simulink model "flux_linkage"  (R2020b)
settings: Solver=VariableStepAuto  StartTime=0.0  StopTime=1  RelTol=1e-3
InitFcn:
  | Rs=0.43;
  | 
  | Lls=0.002
  | 
  | Rr=0.816;
  | 
  | Llr=0.002
  | 
  | Lm=0.6931;
  | 
  | 
  | J=0.085;
  | np=2;
  | 
  | Ts=1e-5;
  | 
  | Udc=600*sqrt(3)
  | Tpwm = 4e-4;
  | 
  | Udc = 2700
  | J = 0.1
  | Llr = 0.006
  | Lls = 0.00116
  | Lm = 0.0254
  | Rr = 0.16
  | Rs = 0.15
  | 
  | Ls = 1.5*Lm+Lls
  | Lr = 1.5*Lm+Llr
  | Tr = Lr/Rr;
  | sigma = (Ls*Lr-Lm*Lm)/Ls/Lr;
model workspace (MAT data in the model file):
  Tsys = 2e-06
  sample_time = 1e-06
libraries: powerlib x17, simulink x3
settings Model: SimulationMode=accelerator  OrderedModelArguments=off  Creator=messer  LastModifiedBy=messer

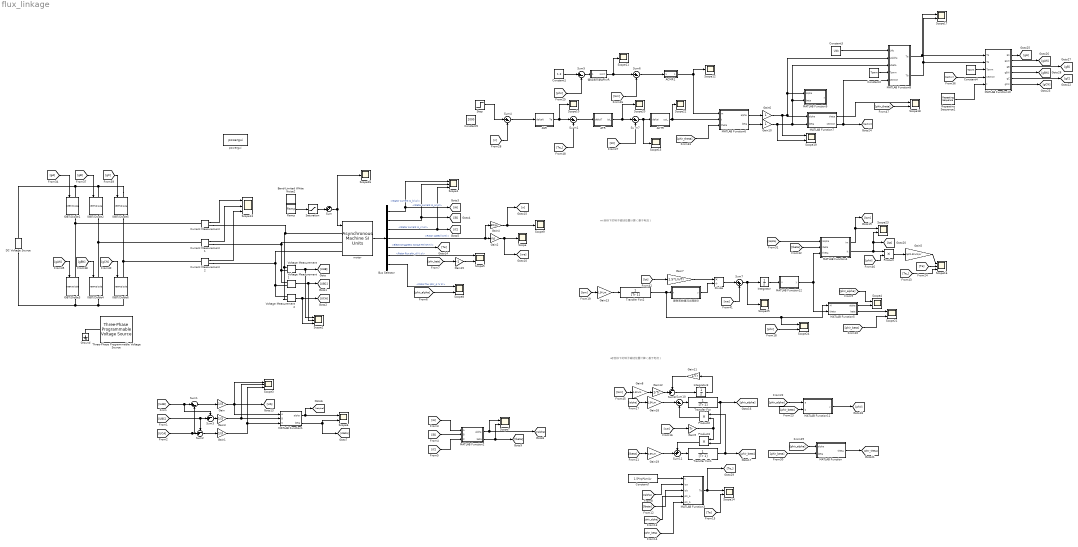
== system flux_linkage ==
  note: αβ坐标下的转子磁链位置计算（基于电流）
  note: mt坐标下的转子磁链位置计算（基于电流）
  ACMR1 : Subsystem
  ACTR : Subsystem
  ASR : Subsystem
  ATR : Subsystem
  Band-Limited White Noise2 : simulink/Sources/Band-Limited White Noise  Cov=[0.0001]  Ts=1e-4  seed=[130341]
  Bus Selector : BusSelector  OutputSignals=Stator measurements.Stator current is_a (A),Stator measurements.Stator current is_b (A),Stator measurements.Stator current is_c (A),Mechanical.Rotor speed (wm),Mechanical.Electromagnetic torque Te (N*m),Rotor measurements.Rotor flux phir_d (V s),Rotor measurements.Rotor flux phir_q (V s)
  Constant1 : Constant  Value=1.2
  Constant2 : Constant  Value=Tpwm
  Constant3 : Constant  Value=Udc
  Constant4 : Constant  Value=Tpwm
  Constant5 : Constant  Value=2000
  Constant7 : Constant  Value=1.5*np*Lm/Lr
  Current Measurement : powerlib/Measurements/Current Measurement  PhasorSimulation=off  OutputType=Complex  PSBequivalent=0
  Current Measurement1 : powerlib/Measurements/Current Measurement  PhasorSimulation=off  OutputType=Complex  PSBequivalent=0
  Current Measurement2 : powerlib/Measurements/Current Measurement  PhasorSimulation=off  OutputType=Complex  PSBequivalent=0
  DC Voltage Source : powerlib/Electrical Sources/DC Voltage Source  Amplitude=Udc  Measurements=None
  Divide : Product  Inputs=*/
  Gain : Gain  Gain=1/3
  Gain1 : Gain  Gain=1/3
  Gain10 : Gain
  Gain11 : Gain  Gain=1/Tr
  Gain12 : Gain  Gain=1/Tr
  Gain{8,13,18..19} (4 alike) : Gain  Gain=1.5*Lm
  Gain15 : Gain  Gain=-1
  Gain2 : Gain  Gain=np
  Gain3 : Gain  Gain=1/3
  Gain4 : Gain  Gain=30/pi
  Gain5 : Gain  Gain=np*1.5*Lm/Lr
  Gain6 : Gain
  Gain7 : Gain  Gain=1.5*Lm/Tr
  Gain9 : Gain  Gain=Tr
  Ground : powerlib/Elements/Ground  LConnTagsString=a
  IGBT/Diode{1..6} (6 alike) : powerlib/Power Electronics/IGBT//Diode  Ron=1e-3  Rs=1e5  Cs=inf  Measurements=on
  Integrator : Integrator  InitialCondition=1e-5
  Integrator3 : Integrator  InitialCondition=1e-5
  MATLAB Function : MATLAB Function  TreatAsAtomicUnit=on
  MATLAB Function1 : MATLAB Function  TreatAsAtomicUnit=on
  MATLAB Function10 : MATLAB Function  TreatAsAtomicUnit=on
  MATLAB Function11 : MATLAB Function  TreatAsAtomicUnit=on
  MATLAB Function12 : MATLAB Function  TreatAsAtomicUnit=on
  MATLAB Function2 : MATLAB Function  TreatAsAtomicUnit=on
  MATLAB Function3 : MATLAB Function  TreatAsAtomicUnit=on
  MATLAB Function4 : MATLAB Function  TreatAsAtomicUnit=on
  MATLAB Function5 : MATLAB Function  TreatAsAtomicUnit=on
  MATLAB Function6 : MATLAB Function  TreatAsAtomicUnit=on
  MATLAB Function7 : MATLAB Function  TreatAsAtomicUnit=on
  MATLAB Function8 : MATLAB Function  TreatAsAtomicUnit=on
  MATLAB Function9 : MATLAB Function  TreatAsAtomicUnit=on
  Product : Product
  Product2 : Product
  Product3 : Product
  Ramp : simulink/Sources/Ramp  slope=100  start=0.15  InitialOutput=5
  Repeating Sequence1 : simulink/Sources/Repeating Sequence  rep_seq_t=[0 Tpwm]  rep_seq_y=[0 Tpwm]
  Saturation : Saturate  UpperLimit=20  LowerLimit=0
  Scope{,9..12,15,20,22,25..26} (10 alike) : Scope
  Scope{1..3,13,16} (5 alike) : Scope  NumInputPorts=3
  Scope{4..8,14,17..19,21,23..24} (12 alike) : Scope  NumInputPorts=2
  Step : Step  Time=0.5  Before=2000  After=3000  SampleTime=0
  Su`m1 : Sum  Inputs=|+-
  Su`m7 : Sum  Inputs=|+-
  Sum : Sum  Inputs=++|
  Sum{1,4..6,10} (5 alike) : Sum  Inputs=|+-
  Sum11 : Sum  Inputs=++|
  Sum2 : Sum  Inputs=-+|
  Sum3 : Sum  Inputs=-+|
  Sum7 : Sum  Inputs=|++
  Sum8 : Sum  Inputs=-+|
  Three-Phase Programmable Voltage Source : powerlib/Electrical Sources/Three-Phase Programmable Voltage Source  PositiveSequence="[380/sqrt(2)  0 50]"  VariationEntity=None  VariationType=Table of time-amplitude pairs  VariationTypeAlt=Step  VariationStep=0.5  VariationRate=10  VariationMagnitude=0.3  VariationFrequency=2  VariationTiming=[1 2]  VariationPhaseA=off  Amplitudes=[1 0.8 1.2 1.0]  TimeValues=[0 0.1 0.15 0.2]  HarmonicGeneration=off  HarmonicA=[3 0.2 -25 0]  HarmonicB=[2 0.15 35 2]  Timing="[0.05  3]"  BusType=swing  Pref=0  Qref=0  Qmin=-inf  Qmax=inf
  Transfer Fcn : TransferFcn  Denominator=[Tr 1]
  Transfer Fcn1 : TransferFcn  Denominator=[Tr 1]
  Transfer Fcn2 : TransferFcn  Denominator=[Tr 1]
  Voltage Measurement : powerlib/Measurements/Voltage Measurement  PhasorSimulation=off  OutputType=Complex  PSBequivalent=0
  Voltage Measurement1 : powerlib/Measurements/Voltage Measurement  PhasorSimulation=off  OutputType=Complex  PSBequivalent=0
  Voltage Measurement2 : powerlib/Measurements/Voltage Measurement  PhasorSimulation=off  OutputType=Complex  PSBequivalent=0
  motor : powerlib/Machines/Asynchronous Machine SI Units  RotorType=Squirrel-cage  PresetModel=No  MechanicalLoad=Torque Tm  ShowDetailedParameters=on  ReferenceFrame=Stationary  Units=SI  MeasurementBus=off  NominalParameters=[562000 2750 135]  Stator=[Rs Lls]  Rotor=[Rr Llr]  Cage1=[0.4155 0.002066]  Cage2=[0.4168 0.0003495]  Lm=Lm  Mechanical=[J 0 np]  PolePairs=2  InitialConditions=[1 0 0 0 0 0 0 0]  SimulateSaturation=off  Saturation=[14.03593122, 27.81365428, 53.79336849, 72.68890987, 97.98006896, 148.6815601, 215.7428561, 302.9841135, 428.7778367 ; 230, 322, 414, 460, 506, 552, 598, 644, 690]  LoadFlowParameters=1492000  TsPowergui=0  TsBlock=-1  IterativeModel=Trapezoidal non iterative  IterativeDiscreteModel=Trapezoidal non iterative  Pmec=1.492e+006
  powergui : powerlib/powergui  Priority=1  SimulationMode=Discrete  SampleTime=Tsys  frequency=60  Iterations=50  frequencyindice=0  Pbase=100e6  ErrMax=1e-4  UnitsV=kV  UnitsW=MW  buscounter=0  FunctionMessages=off  echomessages=off  EnableUseOfTLC=off  CurrentSourceSwitches=off  DisableSnubberDevices=off  DisableRonSwitches=off  DisableVfSwitches=off  DisplayEquations=off  AutomaticDiscreteSolvers=off  SolverType=Tustin/Backward Euler (TBE)  Interpol=off  ExternalGateDelay=off  methode=off  Ts=100  x0status=blocks  SPID=on  SwTol=0  HookPort=off  NonlinearTolerance=1e-4  nMaxIteration=100  ContinueOnMaxIteration=off  RestoreLinks=warning  ResistiveCurrentMeasurement=off  Frange=[0:2:500]  Ylog=off  Xlog=on  ShowGrid=off  save=off  variable=ZData  structure=0  ZoomFFT=off  StartTime=0.0  cycles=1  DisplayStyle=1  fundamental=60  FreqAxis=off  MaxFrequency=1000  frequencyindicesteady=1  RmsSteady=1  display=off
  磁链调节器APhirR : Subsystem
  避免初始情况出现除0 : MATLAB Function  TreatAsAtomicUnit=on
  wires:
  Bus Selector/4 -> Gain4/1, Gain2/1  "<Rotor speed (wm)>"
  Bus Selector/2 -> Scope1/2, [iB]  "<Stator current is_b (A)>"
  Bus Selector/5 -> [Te]  "<Electromagnetic torque Te (N*m)>"
  Saturation/1 -> Sum/2
  Bus Selector/1 -> [iA], Scope1/1  "<Stator current is_a (A)>"
  motor/1 -> Bus Selector/1
  Bus Selector/3 -> Scope1/3, [iC]  "<Stator current is_c (A)>"
  Ramp/1 -> Saturation/1
  Voltage Measurement1/1 -> [UBC], Scope2/2
  Voltage Measurement/1 -> Scope2/1, [UAB]
  Voltage Measurement2/1 -> [UCA], Scope2/3
  [UAB] -> Sum3/1, Sum1/1
  [UCA] -> Sum1/2, Sum2/2
  Sum1/1 -> Gain/1
  [UBC] -> Sum2/1, Sum3/2
  Sum2/1 -> Gain1/1
  Sum3/1 -> Gain3/1
  Gain3/1 -> MATLAB Function1/2(B), Scope3/2
  Gain/1 -> MATLAB Function1/1(A), [UA], Scope3/1
  Gain1/1 -> MATLAB Function1/3(C), Scope3/3
  Sum/1 -> Scope26/1, motor/1
  MATLAB Function1/1(alpha) -> [Ualpha], Scope6/1
  MATLAB Function1/2(beta) -> [Ubeta], Scope6/2
  MATLAB Function2/2(beta) -> [Ibeta], Scope7/2
  [iB] -> MATLAB Function2/2(B)
  MATLAB Function2/1(alpha) -> Scope7/1, [Ialpha]
  [phir_alpha] -> Scope8/2
  [phir_beta] -> Gain15/1
  Gain15/1 -> Scope5/2
  Bus Selector/6 -> Scope5/1  "<Rotor flux phir_d (V s)>"
  Bus Selector/7 -> Scope8/1  "<Rotor flux phir_q (V s)>"
  Gain2/1 -> [we], Scope/1
  [iA] -> MATLAB Function2/1(A)
  [iC] -> MATLAB Function2/3(C)
  Constant7/1 -> MATLAB Function3/1(c)
  [Ialpha] -> MATLAB Function3/2(isa)
  [Ibeta] -> MATLAB Function3/3(isb)
  [phir_alpha] -> MATLAB Function3/4(phi_a)
  [phir_beta] -> MATLAB Function3/5(phi_b)
  MATLAB Function3/1(Te) -> [Te_], Scope14/1
  [Te] -> Scope14/2
  Gain4/1 -> [n], Scope9/1
  Current Measurement1/1 -> Scope13/2
  Current Measurement2/1 -> Scope13/3
  Current Measurement/1 -> Scope13/1
  [Ialpha] -> MATLAB Function4/1(Ialpha)
  [Ibeta] -> MATLAB Function4/2(Ibeta)
  MATLAB Function4/2(It) -> Scope23/2, [Ist], Product/1
  Product/1 -> Gain5/1
  Gain5/1 -> Scope16/1
  [Te] -> Scope16/2
  Constant1/1 -> Sum5/1
  [phir] -> Sum5/2
  Sum5/1 -> 磁链调节器APhirR/1(" ")
  MATLAB Function4/1(Im) -> [Ism], Scope23/1
  Repeating Sequence1/1 -> MATLAB Function10/5(t)
  [section] -> MATLAB Function10/4(section)
  Constant3/1 -> MATLAB Function8/1(Udc)
  MATLAB Function8/1(Ta) -> MATLAB Function10/1(Ta), Scope17/1
  MATLAB Function8/2(Tb) -> Scope17/2, MATLAB Function10/2(Tb)
  Constant2/1 -> MATLAB Function8/4(Tpwm)
  MATLAB Function7/1(theta) -> Scope18/1
  Constant4/1 -> MATLAB Function10/3(Tpwm)
  MATLAB Function7/2(section) -> [section], MATLAB Function8/5(section)
  [gA] -> IGBT/Diode1/1
  [gAN] -> IGBT/Diode3/1
  [gB] -> IGBT/Diode2/1
  [gBN] -> IGBT/Diode4/1
  [gC] -> IGBT/Diode5/1
  [gCN] -> IGBT/Diode6/1
  Su`m7/1 -> Scope15/1, ACTR/1(deltaI)
  [Ist] -> Gain7/1
  Gain7/1 -> Divide/1
  Divide/1 -> Sum7/1
  [we] -> Sum7/2
  Sum7/1 -> Scope25/1, Integrator/1
  ACTR/1(ust_) -> MATLAB Function6/2(t), Scope22/1
  [Ism] -> Gain8/1
  [phir] -> Product/2
  Gain8/1 -> Gain12/1
  Integrator3/1 -> Gain11/1
  Sum8/1 -> Integrator3/1
  [n] -> Sum4/2
  [Ist] -> Su`m7/2
  [Ism] -> Sum6/2
  Integrator/1 -> MATLAB Function12/1(x)
  磁链调节器APhirR/1(ism*) -> Scope11/1, Sum6/1
  [phir_theta] -> Scope18/2
  [phir_theta] -> MATLAB Function6/3(theta)
  Sum6/1 -> ACMR1/1("  ")
  ASR/1(Te) -> Scope10/1, Su`m1/1
  Sum4/1 -> ASR/1(deltaN)
  [Te_] -> Su`m1/2
  Su`m1/1 -> ATR/1(deltaT)
  ATR/1(ist_) -> Scope20/1, Su`m7/1
  ACMR1/1(" ") -> Scope12/1, MATLAB Function6/1(m)
  Gain6/1 -> Scope19/1, MATLAB Function7/1(alpha), MATLAB Function8/2(Ualpha), MATLAB Function9/1(alpha)
  Gain10/1 -> Scope19/2, MATLAB Function8/3(Ubeta), MATLAB Function9/2(beta), MATLAB Function7/2(beta)
  MATLAB Function6/1(alpha) -> Gain6/1
  MATLAB Function6/2(beta) -> Gain10/1
  MATLAB Function10/2(gAN) -> [gAN]
  MATLAB Function10/1(gA) -> [gA]
  MATLAB Function10/3(gB) -> [gB]
  MATLAB Function10/4(gBN) -> [gBN]
  MATLAB Function10/5(gC) -> [gC]
  MATLAB Function10/6(gCN) -> [gCN]
  Step/1 -> Sum4/1
  Gain11/1 -> Sum8/1
  Gain12/1 -> Sum8/2
  Sum10/1 -> Transfer Fcn/1
  Gain18/1 -> Sum10/1
  Sum11/1 -> Transfer Fcn1/1
  Product2/1 -> Sum10/2
  Gain19/1 -> Sum11/2
  [Ibeta] -> Gain19/1
  [Ialpha] -> Gain18/1
  Transfer Fcn/1 -> Product3/2, [phir_alpha]
  [we] -> Gain9/1
  Product3/1 -> Sum11/1
  Gain9/1 -> Product3/1, Product2/2
  Transfer Fcn1/1 -> Product2/1, [phir_beta]
  [phir_alpha] -> MATLAB Function11/1(a)
  [phir_beta] -> MATLAB Function11/2(b)
  [phir_beta] -> MATLAB Function/2(beta)
  [phir_alpha] -> MATLAB Function/1(alpha)
  MATLAB Function11/1(y) -> [phir]
  MATLAB Function/1(theta) -> [phir_theta]
  MATLAB Function12/1(y) -> MATLAB Function4/3(theta), MATLAB Function5/2(theta)
  MATLAB Function5/1(alpha) -> Scope4/2
  [phir_alpha] -> Scope4/1
  MATLAB Function5/2(beta) -> Scope21/1
  [phir_beta] -> Scope21/2
  [phir] -> Scope24/2
  [Ism] -> Gain13/1
  Gain13/1 -> Transfer Fcn2/1
  避免初始情况出现除0/1(y) -> Divide/2
  Transfer Fcn2/1 -> Scope24/1, MATLAB Function5/1(M), 避免初始情况出现除0/1(x)
  [Te_] -> Scope16/3
  connections:
  Voltage Measurement1/LConn1 -- Voltage Measurement/LConn2 -- motor/LConn2 -- Current Measurement1/RConn1
  Voltage Measurement2/LConn1 -- Voltage Measurement1/LConn2 -- Current Measurement2/RConn1 -- motor/LConn3
  Voltage Measurement/LConn1 -- Voltage Measurement2/LConn2 -- Current Measurement/RConn1 -- motor/LConn1
  Ground/LConn1 -- Three-Phase Programmable Voltage Source/LConn1
  IGBT/Diode2/RConn1 -- Current Measurement1/LConn1 -- IGBT/Diode4/LConn1
  IGBT/Diode5/LConn1 -- DC Voltage Source/RConn1 -- IGBT/Diode1/LConn1 -- IGBT/Diode2/LConn1
  IGBT/Diode5/RConn1 -- IGBT/Diode6/LConn1 -- Current Measurement2/LConn1
  IGBT/Diode3/RConn1 -- DC Voltage Source/LConn1 -- IGBT/Diode4/RConn1 -- IGBT/Diode6/RConn1
  IGBT/Diode1/RConn1 -- IGBT/Diode3/LConn1 -- Current Measurement/LConn1

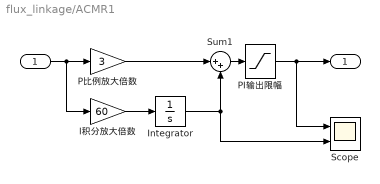
== system flux_linkage/ACMR1 ==
  "  " : Inport
  Integrator : Integrator
  I积分放大倍数 : Gain  Gain=60
  PI输出限幅 : Saturate  UpperLimit=Udc/sqrt(6)  LowerLimit=-Udc/sqrt(6)
  P比例放大倍数 : Gain  Gain=3
  Scope : Scope  NumInputPorts=2
  Sum1 : Sum  Inputs=|++
  " " : Outport  VectorParamsAs1DForOutWhenUnconnected=off
  wires:
  Sum1/1 -> PI输出限幅/1
  PI输出限幅/1 -> " "/1, Scope/1
  P比例放大倍数/1 -> Sum1/1
  I积分放大倍数/1 -> Integrator/1
  "  "/1 -> I积分放大倍数/1, P比例放大倍数/1
  Integrator/1 -> Scope/2, Sum1/2

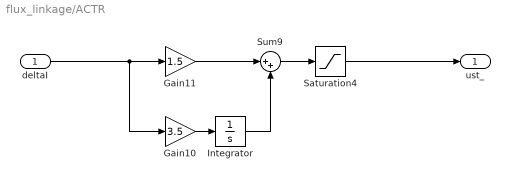
== system flux_linkage/ACTR ==
  deltaI : Inport
  Gain10 : Gain  Gain=3.5
  Gain11 : Gain  Gain=1.5
  Integrator : Integrator
  Saturation4 : Saturate  UpperLimit=Udc/sqrt(3)  LowerLimit=-Udc/sqrt(3)
  Sum9 : Sum  Inputs=|++
  ust_ : Outport
  wires:
  Gain10/1 -> Integrator/1
  Sum9/1 -> Saturation4/1
  Integrator/1 -> Sum9/2
  Saturation4/1 -> ust_/1
  deltaI/1 -> Gain10/1, Gain11/1
  Gain11/1 -> Sum9/1

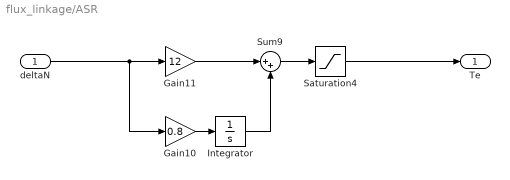
== system flux_linkage/ASR ==
  deltaN : Inport
  Gain10 : Gain  Gain=0.8
  Gain11 : Gain  Gain=12
  Integrator : Integrator
  Saturation4 : Saturate  UpperLimit=300  LowerLimit=-300
  Sum9 : Sum  Inputs=|++
  Te : Outport
  wires:
  Gain11/1 -> Sum9/1
  deltaN/1 -> Gain11/1, Gain10/1
  Saturation4/1 -> Te/1
  Gain10/1 -> Integrator/1
  Sum9/1 -> Saturation4/1
  Integrator/1 -> Sum9/2

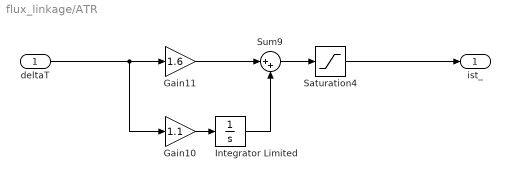
== system flux_linkage/ATR ==
  deltaT : Inport
  Gain10 : Gain  Gain=1.1
  Gain11 : Gain  Gain=1.6
  Integrator Limited : Integrator  LimitOutput=on  UpperSaturationLimit=500  LowerSaturationLimit=-500
  Saturation4 : Saturate  UpperLimit=300  LowerLimit=-300
  Sum9 : Sum  Inputs=|++
  ist_ : Outport
  wires:
  Gain10/1 -> Integrator Limited/1
  Sum9/1 -> Saturation4/1
  Integrator Limited/1 -> Sum9/2
  Saturation4/1 -> ist_/1
  deltaT/1 -> Gain10/1, Gain11/1
  Gain11/1 -> Sum9/1

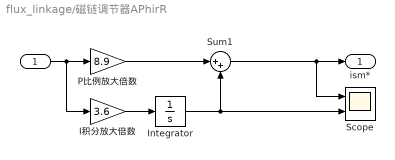
== system flux_linkage/磁链调节器APhirR ==
  " " : Inport
  Integrator : Integrator
  I积分放大倍数 : Gain  Gain=3.6
  P比例放大倍数 : Gain  Gain=8.9
  Scope : Scope  NumInputPorts=2
  Sum1 : Sum  Inputs=|++
  ism* : Outport  VectorParamsAs1DForOutWhenUnconnected=off
  wires:
  P比例放大倍数/1 -> Sum1/1
  " "/1 -> I积分放大倍数/1, P比例放大倍数/1
  Sum1/1 -> ism*/1, Scope/1
  I积分放大倍数/1 -> Integrator/1
  Integrator/1 -> Scope/2, Sum1/2

== matlab function flux_linkage/MATLAB Function7 ==
  data: theta output; alpha input; section output; beta input
function [theta, section] = fcn(alpha, beta)

if(beta >=0)
    if(alpha == 0)
        theta = pi/2;
    elseif(alpha >0)
        theta = atan(beta/alpha);
    else
        theta = pi + atan(beta/alpha);
    end
else
    if(alpha == 0)
        theta = 1.5*pi;
    elseif(alpha > 0)
        theta = 2*pi + atan(beta/alpha);
    else
        theta = pi + atan(beta/alpha);
    end
end


k = sqrt(3);
if(beta > 0)
    if(beta < alpha*k)
        section = 0;
    elseif(beta <= -alpha*k)
        section = 2;
    else
        section = 1;
    end
    
else
    if(beta >= -alpha*k)
        section = 5;
    elseif(beta > alpha*k)
        section = 3;
    else
        section = 4;
    end
end

== matlab function flux_linkage/MATLAB Function8 ==
  data: Udc input; Ta output; Ualpha input; Ubeta input; Tpwm input; section input; Tb output
function [Ta, Tb] = fcn(Udc, Ualpha, Ubeta,  Tpwm, section)

theta = section*pi/3;
Ualpha_ = cos(theta) * Ualpha + sin(theta) * Ubeta;
Ubeta_ = -sin(theta) * Ualpha + cos(theta) * Ubeta;

% Uref,
% if(Uref >= Udc / sqrt(3))
%     Uref = Udc / sqrt(3);
% end
% theta = theta - section*pi/3;
% 
% Ta = sqrt(3)*Uref/Udc*sin(pi/3 - theta) * Tpwm;
% Tb = sqrt(3)*Uref/Udc * sin(theta) * Tpwm;

Ta = (Ualpha_ - Ubeta_/sqrt(3) ) * 1.5 * Tpwm / Udc;
Tb = sqrt(3) * Ubeta_ / Udc * Tpwm;

== matlab function flux_linkage/MATLAB Function9 ==
  data: alpha input; y output; beta input
function y = fcn(alpha, beta)

y = sqrt(alpha*alpha + beta*beta);

== matlab function flux_linkage/MATLAB Function ==
  data: theta output; alpha input; beta input
function theta = fcn(alpha, beta)

if(beta >=0)
    if(alpha == 0)
        theta = pi/2;
    elseif(alpha >0)
        theta = atan(beta/alpha);
    else
        theta = pi + atan(beta/alpha);
    end
else
    if(alpha == 0)
        theta = 1.5*pi;
    elseif(alpha > 0)
        theta = 2*pi + atan(beta/alpha);
    else
        theta = pi + atan(beta/alpha);
    end
end

== matlab function flux_linkage/MATLAB Function12 ==
  data: y output; x input
function y = fcn(x)

y = mod(x, 2*pi);

== matlab function flux_linkage/避免初始情况出现除0 ==
  data: y output; x input
function y = fcn(x)

if(x==0)
    y = 1;
else
    y = x;
end

== matlab function flux_linkage/MATLAB Function1 ==
  data: A input; alpha output; B input; C input; beta output
function [alpha, beta] = fcn(A, B, C)
k = 2/ 3;
alpha = k * (A - 0.5*B - 0.5*C);
beta = k * sqrt(3) / 2 * (B - C);

== matlab function flux_linkage/MATLAB Function5 ==
  data: alpha output; M input; theta input; beta output
function [alpha, beta] = fcn(M, theta)

alpha = M * cos(theta);
beta = M * sin(theta);

== matlab function flux_linkage/MATLAB Function2 ==
  data: A input; alpha output; B input; C input; beta output
function [alpha, beta] = fcn(A, B, C)
k = 2/ 3;
alpha = k * (A - 0.5*B - 0.5*C);
beta = k * sqrt(3) / 2 * (B - C);

== matlab function flux_linkage/MATLAB Function3 ==
  data: c input; Te output; isa input; isb input; phi_a input; phi_b input
function Te = fcn(c, isa, isb, phi_a, phi_b)
Te = c *( isb * phi_a - isa * phi_b);

== matlab function flux_linkage/MATLAB Function4 ==
  data: Im output; Ialpha input; Ibeta input; theta input; It output
function [Im, It] = fcn(Ialpha, Ibeta, theta)

Im = Ialpha * cos(theta) + Ibeta * sin(theta);
It = -Ialpha * sin(theta) + Ibeta * cos(theta);

== matlab function flux_linkage/MATLAB Function11 ==
  data: y output; a input; b input
function y = fcn(a, b)

y = sqrt(a*a + b*b);

== matlab function flux_linkage/MATLAB Function6 ==
  data: alpha output; m input; t input; theta input; beta output
function [alpha, beta] = fcn(m, t, theta)

alpha = cos(theta) * m - sin(theta) * t;
beta = sin(theta) * m + cos(theta) * t;

== matlab function flux_linkage/MATLAB Function10 ==
  data: Ta input; gA output; Tb input; Tpwm input; section input; t input; gAN output; gB output; gBN output; gC output; gCN output
function [gA,gAN, gB, gBN, gC, gCN]  = fcn(Ta, Tb, Tpwm, section, t)

gA = (1==1);
gB = (1==1);
gC = (1==1);

T0 = Tpwm - Ta - Tb;

% 七段式 SPWM，扇区 0~5，对应6个扇区

if(mod(section, 2) == 0 ) % 0、2、4扇区
    t1 = T0/4;
    t2 = t1 + Ta / 2;
    t3 = t2 + Tb / 2;
    t4 = t3 + T0 / 2;
    t5 = t4 + Tb / 2;
    t6 = t5 + Ta / 2;
    
    if(section == 0)
        gA = (t >=t1 && t <=t6);
        gB = (t >=t2 && t <= t5);
        gC = (t >=t3 && t <= t4);
    elseif(section == 2)
        gB = (t >=t1 && t <=t6);
        gC = (t >=t2 && t <= t5);
        gA = (t >=t3 && t <= t4);
    else
        gC = (t >=t1 && t <=t6);
        gA = (t >=t2 && t <= t5);
        gB = (t >=t3 && t <= t4);
    end
else
    t1 = T0/4;
    t2 = t1 + Tb / 2;
    t3 = t2 + Ta / 2;
    t4 = t3 + T0 / 2;
    t5 = t4 + Ta / 2;
    t6 = t5 + Tb / 2;
    
    if(section == 1)
        gB = (t >=t1 && t <=t6);
        gA = (t >=t2 && t <= t5);
        gC = (t >=t3 && t <= t4);
    elseif(section == 3)
        gC = (t >=t1 && t <=t6);
        gB = (t >=t2 && t <= t5);
        gA = (t >=t3 && t <= t4);
    else
        gA = (t >=t1 && t <=t6);
        gC = (t >=t2 && t <= t5);
        gB = (t >=t3 && t <= t4);        
    end
    
end

% gA = gA;
% gB = gB;
% gC = gC;

gAN = ~gA;
gBN = ~gB;
gCN = ~gC;
% g = [gA, 1-gA, gB, 1-gB, gC, 1-gC];
